simulink model "sampleModel1610"  (R2023a)
settings: Solver=VariableStepAuto  StartTime=0.0  StopTime=10.0  RelTol=1e-3
libraries: hdlsllib x6, simulink x4
settings Model: Creator=user1  LastModifiedBy=user1

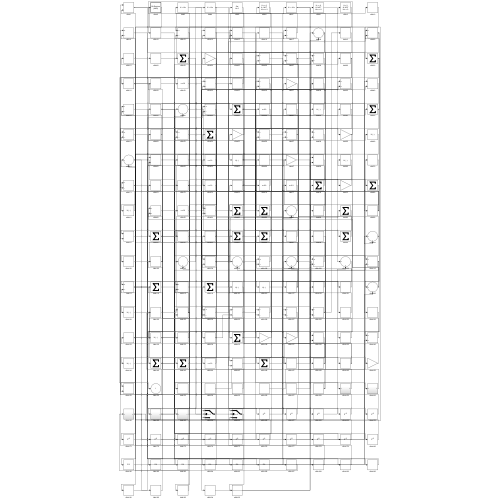
[thumbnail: Simulink's stored preview of the top-level diagram]
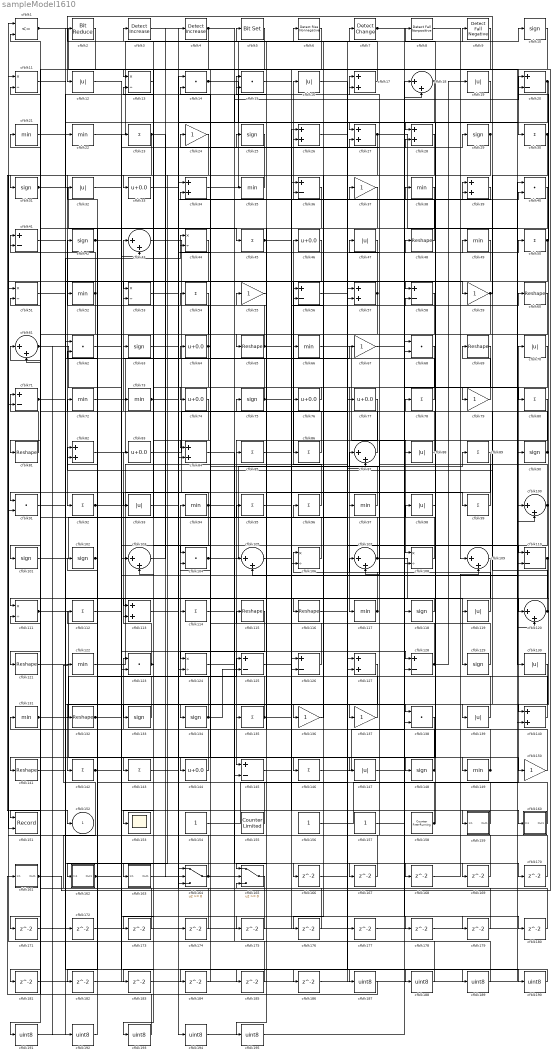
== system sampleModel1610 ==
  cfblk1 : RelationalOperator  Operator=<=  OutDataTypeStr=boolean  InputSameDT=off
  cfblk{10,25,29,31,42,63,75,90,101..102,118,129,133..134,148} (15 alike) : Signum
  cfblk{18,43,61,87,100,103,105,107,109,120} (10 alike) : Sum  Inputs=|++
  cfblk{14..15,40,62,68,91,104,123,138} (9 alike) : DotProduct  OutDataTypeStr=Inherit: Inherit via internal rule
  cfblk{11,13,44,51,53,106,108,111,124} (9 alike) : Product  Inputs=*/  RndMeth=Zero  SaturateOnIntegerOverflow=on
  cfblk{20,36,41,56,58,71,110,125..126,128,145} (11 alike) : Sum  Inputs=+-
  cfblk{23,30,45,50,54,78,80,85..86,89,92,95..96,99,112,114,135,142..143,146} (20 alike) : Sum  Inputs=+
  cfblk{17,26..28,34,39,57,82,84,113,127,140} (12 alike) : Sum
  cfblk{48,60,65,69,81,115..116,121,132,141} (10 alike) : Reshape
  cfblk{21..22,35,38,49,52,66,72..73,94,97,117,122,131,149} (15 alike) : MinMax
  cfblk{12,16,19,32,47,70,88,93,98,119,130,139,147} (13 alike) : Abs  SaturateOnIntegerOverflow=off
  cfblk{24,37,55,59,67,79,136..137,150} (9 alike) : Gain
  cfblk{33,46,64,74,76..77,83,144} (8 alike) : Bias  Bias=0.0  SaturateOnIntegerOverflow=off
  cfblk151 : Record  FileSettingsInternal="{\"entries\":[{\"content\":{\"excelSettings\":{\"content\":{},\"type\":\"Streamout.ExcelSettings\"}},\"type\":\"Streamout.FileSettingStorage\",\"uuid\":\"\"}],\"packageUris\":[\"http:\\/\\/schema.mathworks.com\\/mf0\\/streamout_blocks\\/R2020a\"],\"version\":\"1.0\"}"  Layout=[1 1]  SignalsInternal="{\"entries\":[{\"content\":{\"signals\":[{\"content\":{\"blockPath\":[],\"dimensions\":[1],\"domain\":\"\",\"lineColor\":\"#a2142f\",\"plots\":[1],\"port\":1,\"signalID\":2314,\"signalName\":\"XY Graph:1\"},\"type\":\"RecordBlkView.Signal\",\"uuid\":\"\"},{\"content\":{\"blockPath\":[],\"dimensions\":[1],\"domain\":\"\",\"lineColor\":\"#139fff\",\"plots\":[1],\"port\":2,\"signalID\":2317,\"signalName\":\"XY Graph:2\"},\"type\":\"RecordBlkView.Signal\",\"uuid\":\"\"}]},\"type\":\"RecordBlkView.InputSignals\",\"uuid\":\"\"}],\"packageUris\":[\"http:\\/\\/schema.mathworks.com\\/mf0\\/streamout_blocks\\/R2020a\"],\"version\":\"1.0\"}"  VisualizationBindings="{\"xyplotplugin\":{\"info\":[{\"series\":[{\"bindingParametersList\":[{\"parameter\":\"X-Axis\",\"signalID\":2314,\"signalName\":\"XY Graph:1\"},{\"parameter\":\"Y-Axis\",\"signalID\":2317,\"signalName\":\"XY Graph:2\"}],\"seriesID\":15744}],\"subplotID\":1}]}}"  CompatibilityTag=XY  st=-1
  cfblk153 : Scope
  cfblk154 : Constant  SampleTime=-1
  cfblk155 : hdlsllib/Sources/Counter Limited  uplimit=7  tsamp=-1
  cfblk156 : Constant  SampleTime=-1
  cfblk157 : Constant  SampleTime=-1
  cfblk158 : hdlsllib/Sources/Counter Free-Running  NumBits=16  tsamp=-1
  cfblk159 : Subsystem
      settings: LibrarySourceBlock=|
      | hdlsllib/Ports &
      | Subsystems/Subsystem
  cfblk160 : Subsystem
      settings: LibrarySourceBlock=|
      | hdlsllib/Ports &
      | Subsystems/Subsystem
  cfblk161 : Subsystem
      settings: LibrarySourceBlock=|
      | hdlsllib/Ports &
      | Subsystems/Subsystem
  cfblk162 : Subsystem
      settings: LibrarySourceBlock=|
      | hdlsllib/Ports &
      | Subsystems/Subsystem
  cfblk163 : Subsystem
      settings: LibrarySourceBlock=|
      | hdlsllib/Ports &
      | Subsystems/Subsystem
  cfblk164 : Switch  SaturateOnIntegerOverflow=off  InputSameDT=off
  cfblk165 : Switch  SaturateOnIntegerOverflow=off  InputSameDT=off
  cfblk{166..186} (21 alike) : Delay  SampleTime=1
  cfblk{187..195} (9 alike) : DataTypeConversion  OutDataTypeStr=uint8  SaturateOnIntegerOverflow=off  RndMeth=Floor
  cfblk2 : hdlsllib/Logic and Bit Operations/Bit Reduce  mode=AND
  cfblk3 : simulink/Logic and Bit Operations/Detect Increase  vinit=0.0  OutDataTypeStr=boolean
      settings: LibrarySourceBlock=|
      | hdlsllib/Logic and Bit
      | Operations/Detect
      | Increase
  cfblk4 : simulink/Logic and Bit Operations/Detect Increase  vinit=0.0  OutDataTypeStr=boolean
      settings: LibrarySourceBlock=|
      | hdlsllib/Logic and Bit
      | Operations/Detect
      | Increase
  cfblk5 : simulink/Logic and Bit Operations/Bit Set  iBit=0
      settings: LibrarySourceBlock=|
      | hdlsllib/Logic and Bit
      | Operations/Bit Set
  cfblk6 : hdlsllib/Logic and Bit Operations/Detect Rise Nonnegative  vinit=0  OutDataTypeStr=boolean
  cfblk7 : simulink/Logic and Bit Operations/Detect Change  vinit=0  OutDataTypeStr=boolean
      settings: LibrarySourceBlock=|
      | hdlsllib/Logic and Bit
      | Operations/Detect
      | Change
  cfblk8 : hdlsllib/Logic and Bit Operations/Detect Fall Nonpositive  vinit=0  OutDataTypeStr=boolean
  cfblk9 : hdlsllib/Logic and Bit Operations/Detect Fall Negative  vinit=0  OutDataTypeStr=boolean
  cfblk152 : Outport  VectorParamsAs1DForOutWhenUnconnected=off
  wires:
  cfblk134/1 -> cfblk94/1, cfblk125/2
  cfblk103/1 -> cfblk4/1
  cfblk81/1 -> cfblk71/1
  cfblk29/1 -> cfblk162/1(In1), cfblk128/2
  cfblk156/1 -> cfblk70/1
  cfblk59/1 -> cfblk12/1, cfblk124/2
  cfblk18/1 -> cfblk104/1, cfblk164/3
  cfblk43/1 -> cfblk145/1
  cfblk89/1 -> cfblk165/1
  cfblk52/1 -> cfblk41/1, cfblk141/1
  cfblk94/1 -> cfblk91/1, cfblk103/2, cfblk17/2
  cfblk23/1 -> cfblk152/1, cfblk164/2
  cfblk71/1 -> cfblk186/1, cfblk191/1
  cfblk54/1 -> cfblk81/1
  cfblk106/1 -> cfblk61/1
  cfblk75/1 -> cfblk43/1, cfblk149/1, cfblk119/1
  cfblk58/1 -> cfblk65/1
  cfblk98/1 -> cfblk148/1
  cfblk27/1 -> cfblk92/1, cfblk100/2
  cfblk140/1 -> cfblk17/1
  cfblk99/1 -> cfblk24/1
  cfblk13/1 -> cfblk143/1
  cfblk163/1(Out1) -> cfblk48/1
  cfblk120/1 -> cfblk75/1, cfblk82/1
  cfblk34/1 -> cfblk10/1
  cfblk154/1 -> cfblk57/1
  cfblk1/1 -> cfblk90/1, cfblk59/1
  cfblk11/1 -> cfblk27/1
  cfblk87/1 -> cfblk11/2
  cfblk90/1 -> cfblk63/1, cfblk44/2, cfblk56/2
  cfblk114/1 -> cfblk35/1
  cfblk96/1 -> cfblk46/1
  cfblk48/1 -> cfblk16/1
  cfblk82/1 -> cfblk36/1
  cfblk65/1 -> cfblk42/1, cfblk110/1, cfblk159/1(In1)
  cfblk117/1 -> cfblk106/1, cfblk15/1
  cfblk148/1 -> cfblk25/1, cfblk78/1
  cfblk21/1 -> cfblk22/1
  cfblk77/1 -> cfblk135/1
  cfblk69/1 -> cfblk117/1
  cfblk149/1 -> cfblk115/1, cfblk123/1
  cfblk150/1 -> cfblk87/1
  cfblk79/1 -> cfblk69/1
  cfblk35/1 -> cfblk33/1
  cfblk157/1 -> cfblk118/1
  cfblk66/1 -> cfblk108/1
  cfblk49/1 -> cfblk86/1
  cfblk139/1 -> cfblk114/1
  cfblk55/1 -> cfblk5/1
  cfblk142/1 -> cfblk160/1(In1), cfblk110/2
  cfblk119/1 -> cfblk107/1
  cfblk123/1 -> cfblk83/1, cfblk113/2, cfblk183/1
  cfblk107/1 -> cfblk129/1, cfblk13/2, cfblk55/1
  cfblk9/1 -> cfblk53/1
  cfblk76/1 -> cfblk74/1
  cfblk100/1 -> cfblk127/2, cfblk47/1
  cfblk128/1 -> cfblk54/1, cfblk19/1
  cfblk95/1 -> cfblk26/1
  cfblk127/1 -> cfblk142/1
  cfblk38/1 -> cfblk153/1
  cfblk30/1 -> cfblk139/1, cfblk120/1
  cfblk111/1 -> cfblk137/1, cfblk67/1, cfblk185/1
  cfblk86/1 -> cfblk41/2
  cfblk42/1 -> cfblk106/2, cfblk175/1
  cfblk36/1 -> cfblk121/1
  cfblk125/1 -> cfblk49/1
  cfblk6/1 -> cfblk134/1
  cfblk64/1 -> cfblk3/1, cfblk84/1, cfblk84/2
  cfblk147/1 -> cfblk108/2
  cfblk88/1 -> cfblk66/1
  cfblk50/1 -> cfblk85/1, cfblk20/2
  cfblk137/1 -> cfblk6/1
  cfblk159/1(Out1) -> cfblk112/1
  cfblk8/1 -> cfblk109/1
  cfblk7/1 -> cfblk80/1, cfblk180/1
  cfblk70/1 -> cfblk136/1
  cfblk53/1 -> cfblk36/2
  cfblk122/1 -> cfblk60/1
  cfblk57/1 -> cfblk56/1, cfblk182/1
  cfblk136/1 -> cfblk96/1
  cfblk101/1 -> cfblk77/1
  cfblk20/1 -> cfblk140/1, cfblk138/1
  cfblk133/1 -> cfblk52/1
  cfblk121/1 -> cfblk145/2
  cfblk46/1 -> cfblk71/2
  cfblk158/1 -> cfblk98/1, cfblk37/1
  cfblk109/1 -> cfblk146/1
  cfblk97/1 -> cfblk64/1
  cfblk102/1 -> cfblk72/1, cfblk32/1
  cfblk61/1 -> cfblk103/1, cfblk172/1
  cfblk110/1 -> cfblk105/2, cfblk176/1
  cfblk165/1 -> cfblk122/1
  cfblk131/1 -> cfblk125/1, cfblk133/1
  cfblk115/1 -> cfblk144/1
  cfblk63/1 -> cfblk150/1
  cfblk91/1 -> cfblk116/1
  cfblk146/1 -> cfblk18/2
  cfblk132/1 -> cfblk43/2, cfblk178/1
  cfblk160/1(Out1) -> cfblk8/1
  cfblk4/1 -> cfblk28/1, cfblk13/1
  cfblk145/1 -> cfblk147/1
  cfblk39/1 -> cfblk34/2
  cfblk56/1 -> cfblk9/1
  cfblk14/1 -> cfblk130/1, cfblk124/1
  cfblk155/1 -> cfblk102/1
  cfblk45/1 -> cfblk97/1, cfblk138/2
  cfblk28/1 -> cfblk76/1
  cfblk161/1(Out1) -> cfblk30/1, cfblk192/1
  cfblk73/1 -> cfblk113/1, cfblk105/1
  cfblk22/1 -> cfblk7/1
  cfblk12/1 -> cfblk73/1
  cfblk78/1 -> cfblk53/2
  cfblk17/1 -> cfblk2/1
  cfblk93/1 -> cfblk39/1
  cfblk130/1 -> cfblk163/1(In1)
  cfblk113/1 -> cfblk39/2
  cfblk83/1 -> cfblk57/2
  cfblk162/1(Out1) -> cfblk23/1, cfblk28/2
  cfblk135/1 -> cfblk29/1, cfblk82/2
  cfblk118/1 -> cfblk111/1
  cfblk25/1 -> cfblk151/1
  cfblk80/1 -> cfblk107/2
  cfblk40/1 -> cfblk132/1
  cfblk47/1 -> cfblk91/2
  cfblk31/1 -> cfblk45/1, cfblk15/2
  cfblk60/1 -> cfblk101/1
  cfblk67/1 -> cfblk79/1
  cfblk124/1 -> cfblk20/1
  cfblk92/1 -> cfblk99/1, cfblk166/1
  cfblk10/1 -> cfblk126/2
  cfblk164/1 -> cfblk111/2, cfblk38/1
  cfblk105/1 -> cfblk40/2
  cfblk19/1 -> cfblk88/1
  cfblk15/1 -> cfblk58/1
  cfblk108/1 -> cfblk26/2
  cfblk104/1 -> cfblk89/1, cfblk50/1
  cfblk144/1 -> cfblk21/1
  cfblk44/1 -> cfblk93/1
  cfblk141/1 -> cfblk44/1
  cfblk24/1 -> cfblk151/2
  cfblk85/1 -> cfblk58/2
  cfblk126/1 -> cfblk14/2
  cfblk129/1 -> cfblk95/1
  cfblk72/1 -> cfblk128/1
  cfblk2/1 -> cfblk31/1
  cfblk166/1 -> cfblk87/2
  cfblk41/1 -> cfblk167/1
  cfblk167/1 -> cfblk11/1
  cfblk16/1 -> cfblk168/1
  cfblk168/1 -> cfblk109/2
  cfblk3/1 -> cfblk169/1
  cfblk169/1 -> cfblk1/1
  cfblk84/1 -> cfblk170/1
  cfblk170/1 -> cfblk27/2
  cfblk138/1 -> cfblk171/1
  cfblk171/1 -> cfblk126/1
  cfblk172/1 -> cfblk18/1
  cfblk74/1 -> cfblk173/1
  cfblk173/1 -> cfblk61/2
  cfblk143/1 -> cfblk174/1
  cfblk174/1 -> cfblk164/1
  cfblk175/1 -> cfblk165/3
  cfblk176/1 -> cfblk34/1
  cfblk26/1 -> cfblk177/1
  cfblk177/1 -> cfblk40/1
  cfblk178/1 -> cfblk140/2
  cfblk112/1 -> cfblk179/1
  cfblk179/1 -> cfblk14/1
  cfblk180/1 -> cfblk1/2
  cfblk5/1 -> cfblk181/1
  cfblk181/1 -> cfblk100/1
  cfblk182/1 -> cfblk123/2
  cfblk183/1 -> cfblk120/2
  cfblk184/1 -> cfblk104/2
  cfblk185/1 -> cfblk165/2
  cfblk186/1 -> cfblk127/1
  cfblk51/1 -> cfblk187/1
  cfblk187/1 -> cfblk161/1(In1)
  cfblk32/1 -> cfblk188/1
  cfblk188/1 -> cfblk51/1
  cfblk116/1 -> cfblk189/1
  cfblk189/1 -> cfblk51/2
  cfblk62/1 -> cfblk190/1
  cfblk190/1 -> cfblk184/1
  cfblk191/1 -> cfblk62/1
  cfblk192/1 -> cfblk62/2
  cfblk68/1 -> cfblk193/1
  cfblk193/1 -> cfblk131/1
  cfblk33/1 -> cfblk194/1
  cfblk194/1 -> cfblk68/1
  cfblk37/1 -> cfblk195/1
  cfblk195/1 -> cfblk68/2

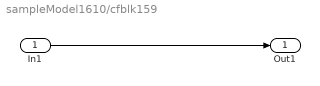
== system sampleModel1610/cfblk159 ==
  In1 : Inport
  Out1 : Outport
  wires:
  In1/1 -> Out1/1

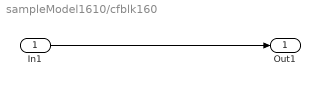
== system sampleModel1610/cfblk160 ==
  In1 : Inport
  Out1 : Outport
  wires:
  In1/1 -> Out1/1

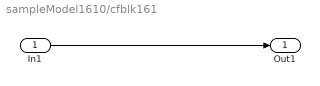
== system sampleModel1610/cfblk161 ==
  In1 : Inport
  Out1 : Outport
  wires:
  In1/1 -> Out1/1

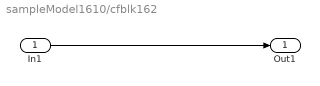
== system sampleModel1610/cfblk162 ==
  In1 : Inport
  Out1 : Outport
  wires:
  In1/1 -> Out1/1

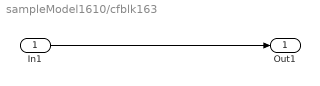
== system sampleModel1610/cfblk163 ==
  In1 : Inport
  Out1 : Outport
  wires:
  In1/1 -> Out1/1
